simulink model "Quadcopter_Model"  (R2021a)
settings: Solver=ode45  StartTime=0.0  StopTime=10.0  RelTol=1e-3
values from neighbouring files (symbols this model uses):
  eta = 1    [Linearize_EOM_V2.m]    (also in Properties_Quad.m)
  g = subs(f,x,x_e)    [Linearize_EOM1.m]    (also in Linearize_EOM_V2.m = 9.8; Properties_Quad.m = 9.8)
  K = Z*S^-1    [Controller_LQR.m]    (also in Linear_Main.mat = [1.22505050327 -0.000706255866309 1.31135338351 2.5356976312; Linearize_EOM1.m; Linearize_EOM_V2.m)
  L = (F2+F3)*dy - (F1+F4)*dy    [Linearize_EOM1.m]    (also in Linearize_EOM_V2.m = 0.114; Properties_Quad.m = 0.155)
  m = 4    [Controller_LQR.m]    (also in Linearize_EOM1.m; Linearize_EOM_V2.m; Properties_Quad.m = 1)
  u_e = zeros(4,1)    [A_and_B_Matricies.m]    (also in Controller_LQR.m; Create_System.m; Linear_Main.mat = [2.45 2.45 2.45 2.45]; Linear_Model.mat = [2.45 2.45 2.45 2.45])
libraries: shared6dof x1
settings Model: Creator=vicen  LastModifiedBy=vicen

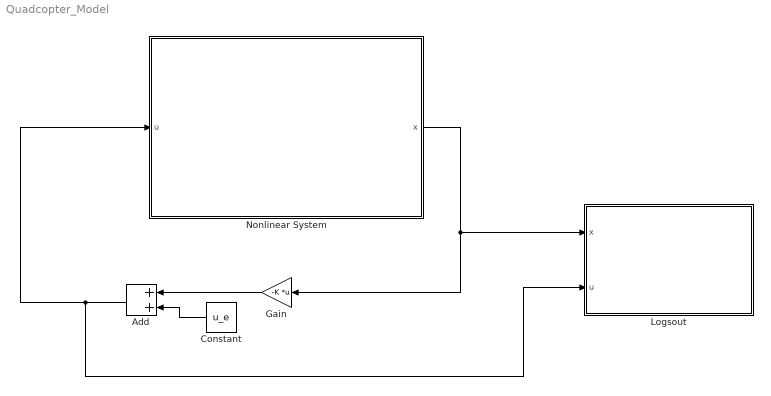
== system Quadcopter_Model ==
  Add : Sum
  Constant : Constant  Value=u_e
  Gain : Gain  Gain=-K  Multiplication=Matrix(K*u)
  Logsout : Subsystem
  Nonlinear System : Subsystem
  wires:
  Add/1 -> Logsout/2(u), Nonlinear System/1(u)
  Gain/1 -> Add/1
  Constant/1 -> Add/2
  Nonlinear System/1(x) -> Gain/1, Logsout/1(x)

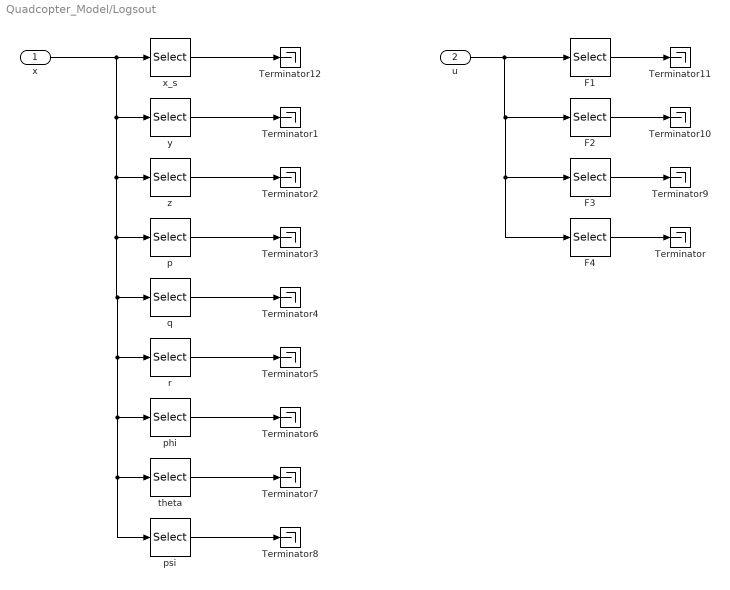
== system Quadcopter_Model/Logsout ==
  x : Inport
  u : Inport  Port=2
  F1 : Selector  InputPortWidth=4  IndexOptions=Index vector (dialog)  Indices=1  OutputSizes=1
  F2 : Selector  InputPortWidth=4  IndexOptions=Index vector (dialog)  Indices=2  OutputSizes=1
  F3 : Selector  InputPortWidth=4  IndexOptions=Index vector (dialog)  Indices=3  OutputSizes=1
  F4 : Selector  InputPortWidth=4  IndexOptions=Index vector (dialog)  Indices=4  OutputSizes=1
  Terminator{,1..12} (13 alike) : Terminator
  p : Selector  InputPortWidth=9  IndexOptions=Index vector (dialog)  Indices=4  OutputSizes=1
  phi : Selector  InputPortWidth=9  IndexOptions=Index vector (dialog)  Indices=7  OutputSizes=1
  psi : Selector  InputPortWidth=9  IndexOptions=Index vector (dialog)  Indices=9  OutputSizes=1
  q : Selector  InputPortWidth=9  IndexOptions=Index vector (dialog)  Indices=5  OutputSizes=1
  r : Selector  InputPortWidth=9  IndexOptions=Index vector (dialog)  Indices=6  OutputSizes=1
  theta : Selector  InputPortWidth=9  IndexOptions=Index vector (dialog)  Indices=8  OutputSizes=1
  x_s : Selector  InputPortWidth=9  IndexOptions=Index vector (dialog)  Indices=1  OutputSizes=1
  y : Selector  InputPortWidth=9  IndexOptions=Index vector (dialog)  Indices=2  OutputSizes=1
  z : Selector  InputPortWidth=9  IndexOptions=Index vector (dialog)  Indices=3  OutputSizes=1
  wires:
  x/1 -> psi/1, theta/1, phi/1, r/1, q/1, p/1, z/1, y/1, x_s/1
  x_s/1 -> Terminator12/1
  y/1 -> Terminator1/1
  z/1 -> Terminator2/1
  p/1 -> Terminator3/1
  q/1 -> Terminator4/1
  r/1 -> Terminator5/1
  phi/1 -> Terminator6/1
  theta/1 -> Terminator7/1
  psi/1 -> Terminator8/1
  u/1 -> F4/1, F3/1, F2/1, F1/1
  F1/1 -> Terminator11/1
  F2/1 -> Terminator10/1
  F3/1 -> Terminator9/1
  F4/1 -> Terminator/1

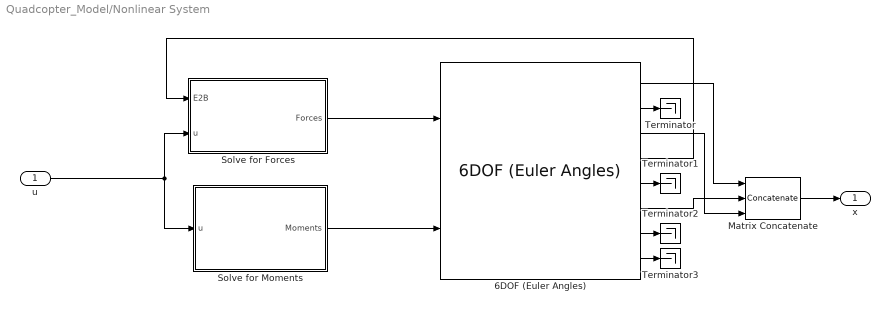
== system Quadcopter_Model/Nonlinear System ==
  u : Inport
  6DOF (Euler Angles) : shared6dof/6DOF (Euler Angles)  units=Metric (MKS)  mtype=Fixed  rep=Euler Angles  xme_0=init.pos_e  Vm_0=init.vel_b  eul_0=init.Euler  pm_0=init.rotation_rates_b  mass_0=m  mass_e=0.5  mass_f=2.0  inertia=I  inertia_e=eye(3)  inertia_f=2*eye(3)  k_quat=1.0  vre_flag=on  abi_flag=off  aMode=0  xme_statename=''  Vm_statename=''  eul_statename=''  quat_statename=''  pm_statename=''  mass_statename=''
      settings: SourceProductBaseCode=AE,PW,DR,MT,UV,VE
  Matrix Concatenate : Concatenate  NumInputs=3  ConcatenateDimension=2
  Solve for Forces : Subsystem
  Solve for Moments : Subsystem
  Terminator{,1..3} (4 alike) : Terminator
  x : Outport
  wires:
  6DOF (Euler Angles)/8 -> Terminator3/1
  6DOF (Euler Angles)/1 -> Matrix Concatenate/1
  6DOF (Euler Angles)/7 -> Terminator2/1
  Matrix Concatenate/1 -> x/1
  u/1 -> Solve for Moments/1(u), Solve for Forces/2(u)
  6DOF (Euler Angles)/6 -> Matrix Concatenate/2
  6DOF (Euler Angles)/3 -> Matrix Concatenate/3
  6DOF (Euler Angles)/5 -> Terminator1/1
  6DOF (Euler Angles)/4 -> Solve for Forces/1(E2B)
  6DOF (Euler Angles)/2 -> Terminator/1
  Solve for Forces/1(Forces) -> 6DOF (Euler Angles)/1
  Solve for Moments/1(Moments) -> 6DOF (Euler Angles)/2

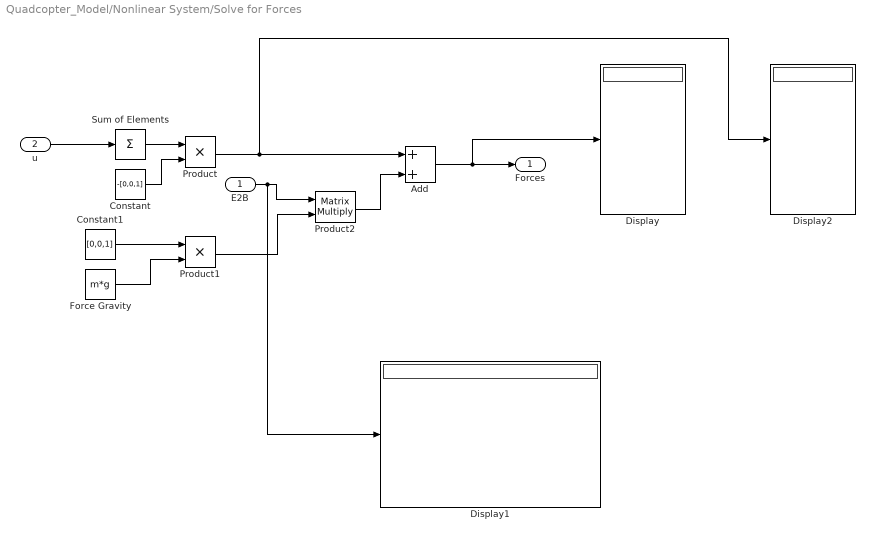
== system Quadcopter_Model/Nonlinear System/Solve for Forces ==
  E2B : Inport
  u : Inport  Port=2
  Add : Sum
  Constant : Constant  Value=-[0,0,1]
  Constant1 : Constant  Value=[0,0,1]
  Display : Display
  Display1 : Display
  Display2 : Display
  Force Gravity : Constant  Value=m*g
  Product : Product
  Product1 : Product
  Product2 : Product  Multiplication=Matrix(*)
  Sum of Elements : Sum  Inputs=+
  Forces : Outport
  wires:
  Product1/1 -> Product2/2
  Product2/1 -> Add/2
  Force Gravity/1 -> Product1/2
  Product/1 -> Display2/1, Add/1
  Constant1/1 -> Product1/1
  Constant/1 -> Product/2
  Sum of Elements/1 -> Product/1
  Add/1 -> Display/1, Forces/1
  u/1 -> Sum of Elements/1
  E2B/1 -> Display1/1, Product2/1

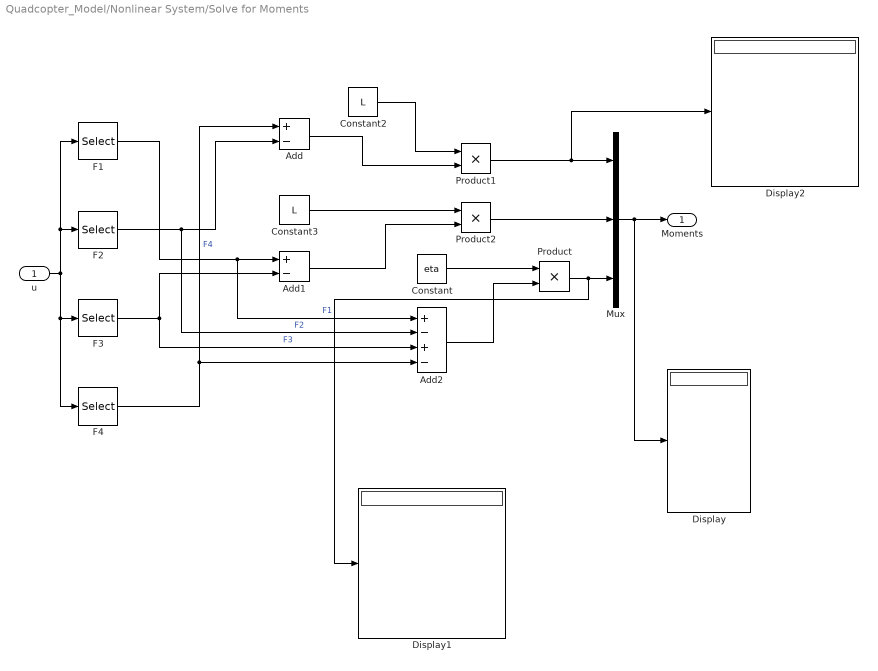
== system Quadcopter_Model/Nonlinear System/Solve for Moments ==
  u : Inport
  Add : Sum  Inputs=+-
  Add1 : Sum  Inputs=+-
  Add2 : Sum  Inputs=+-+-
  Constant : Constant  Value=eta
  Constant2 : Constant  Value=L
  Constant3 : Constant  Value=L
  Display : Display
  Display1 : Display
  Display2 : Display
  F1 : Selector  InputPortWidth=4  IndexOptions=Index vector (dialog)  Indices=1  OutputSizes=1
  F2 : Selector  InputPortWidth=4  IndexOptions=Index vector (dialog)  Indices=2  OutputSizes=1
  F3 : Selector  InputPortWidth=4  IndexOptions=Index vector (dialog)  Indices=3  OutputSizes=1
  F4 : Selector  InputPortWidth=4  IndexOptions=Index vector (dialog)  Indices=4  OutputSizes=1
  Mux : Mux  Inputs=3
  Product : Product
  Product1 : Product
  Product2 : Product
  Moments : Outport
  wires:
  Mux/1 -> Display/1, Moments/1
  u/1 -> F1/1, F2/1, F4/1, F3/1
  F2/1 -> Add2/2, Add/2  "F2"
  F3/1 -> Add2/3, Add1/2  "F3"
  F4/1 -> Add2/4, Add/1  "F4"
  Constant/1 -> Product/1
  Constant2/1 -> Product1/1
  Product1/1 -> Display2/1, Mux/1
  Product2/1 -> Mux/2
  Constant3/1 -> Product2/1
  Add/1 -> Product1/2
  Add1/1 -> Product2/2
  F1/1 -> Add2/1, Add1/1  "F1"
  Product/1 -> Display1/1, Mux/3
  Add2/1 -> Product/2
